simulink model "mrefrobotarm_modified_previous_y_previous_u_previous_ref_Thao"  (R2018b)
settings: Solver=FixedStepAuto  StartTime=0.0  StopTime=10  RelTol=1e-3  AbsTol=1e-6
undefined symbols (not defined in the file or in its folder): sfunxy2
libraries: neural x668, simulink x1
(part 15 of 21)

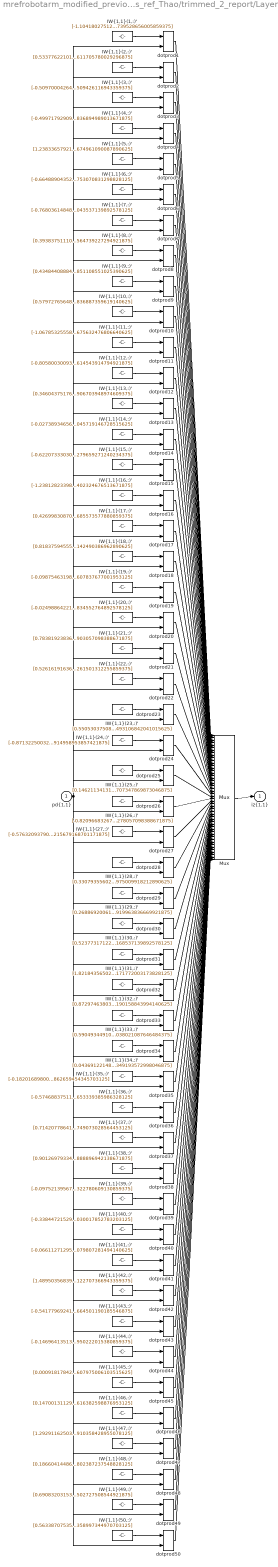
== system mrefrobotarm_modified_previous_y_previous_u_previous_ref_Thao/trimmed_2_report/Layer 1/IW{1,1} ==
  "pd{1,1}" : Inport  PortDimensions=10
      mask Display: e = 0.06;c1 = [120 230 180]/255;c2 = ([120 230 180]+0)/(256+128);c3 = ([120 230 180]+128)/(256+128);patch([0 1 1 0],[0 0 1 1],c1);patch([0 1 1 1-e 1-e 0+e],[0 0 1 1-e 0+e 0+e],c2);patch([0 0 1 1-e 0+e 0+e],[0 1 1 1-e 1-e 0+e],c3);plot([0 1 1 0 0],[0 0 1 1 0]);
  "IW{1,1}(1,:)'" : Constant  Value=[-1.104180275120626220086705870926380157470703125;1.3041448994089861468381741360644809901714324951171875;0.32348674993063841753837550641037523746490478515625;0.0954597345916509965046969909963081590831279754638671875;0.58458283056964244206454850427689962089061737060546875;0.12370355290676347814748936571049853228032588958740234375;-0.360929014481330023844662946430617012083530426025390625;-0.51372399216258501919440959682106040418148040771484375;0.43363839042661889155994003886007703840732574462890625;-0.78302167032477354435826555345556698739528656005859375]
      mask Display: e = 0.06;c1 = [120 150 230]/255;c2 = ([120 150 230]+0)/383;c3 = ([120 150 230]+128)/383;patch([0 1 1 0],[0 0 1 1],c1);patch([0 1 1 1-e 1-e 0+e],[0 0 1 1-e 0+e 0+e],c2);patch([0 0 1 1-e 0+e 0+e],[0 1 1 1-e 1-e 0+e],c3);plot([0 1 1 0 0],[0 0 1 1 0]);disp('Weights');
  "IW{1,1}(10,:)'" : Constant  Value=[0.57972765648551993766801615493022836744785308837890625;0.56702883929374958693614416915806941688060760498046875;0.73417648924284450995259021510719321668148040771484375;-0.545536348624968692178072160459123551845550537109375;-0.85212502298467096562006872773054055869579315185546875;0.9171593407120699481538395048119127750396728515625;0.486441425317741593659093268797732889652252197265625;-1.19193592499658951311403143336065113544464111328125;-0.34835369047706132850095173125737346708774566650390625;-0.277702966436770781744058922413387335836887359619140625]
      mask Display: e = 0.06;c1 = [120 150 230]/255;c2 = ([120 150 230]+0)/383;c3 = ([120 150 230]+128)/383;patch([0 1 1 0],[0 0 1 1],c1);patch([0 1 1 1-e 1-e 0+e],[0 0 1 1-e 0+e 0+e],c2);patch([0 0 1 1-e 0+e 0+e],[0 1 1 1-e 1-e 0+e],c3);plot([0 1 1 0 0],[0 0 1 1 0]);disp('Weights');
  "IW{1,1}(11,:)'" : Constant  Value=[-1.067853255585921257164727649069391191005706787109375;0.73612625892691163631553763480042107403278350830078125;0.6564643621126766692697174221393652260303497314453125;0.2467046979952456087215040270166355185210704803466796875;-0.99137542418344748451630721319816075265407562255859375;-0.265054621061350637045705980199272744357585906982421875;0.086378144705514525725220664753578603267669677734375;-0.5348493447178370718830819896538741886615753173828125;0.3771915850785896306973654645844362676143646240234375;0.617872935716521798354960992583073675632476806640625]
      mask Display: e = 0.06;c1 = [120 150 230]/255;c2 = ([120 150 230]+0)/383;c3 = ([120 150 230]+128)/383;patch([0 1 1 0],[0 0 1 1],c1);patch([0 1 1 1-e 1-e 0+e],[0 0 1 1-e 0+e 0+e],c2);patch([0 0 1 1-e 0+e 0+e],[0 1 1 1-e 1-e 0+e],c3);plot([0 1 1 0 0],[0 0 1 1 0]);disp('Weights');
  "IW{1,1}(12,:)'" : Constant  Value=[-0.80580030093587506900831840539467521011829376220703125;0.76359779607282451951988377913949079811573028564453125;-1.22625268437045331637591516482643783092498779296875;-0.052095597808536391049027969302187557332217693328857421875;-0.65232187763079341191740923022734932601451873779296875;-1.2613588707820095891065648174844682216644287109375;0.48668873664058853734104559407569468021392822265625;0.431726260476050394121472209008061327040195465087890625;-0.98679278575181406107930115467752330005168914794921875;-0.710264778984373901238313919748179614543914794921875]
      mask Display: e = 0.06;c1 = [120 150 230]/255;c2 = ([120 150 230]+0)/383;c3 = ([120 150 230]+128)/383;patch([0 1 1 0],[0 0 1 1],c1);patch([0 1 1 1-e 1-e 0+e],[0 0 1 1-e 0+e 0+e],c2);patch([0 0 1 1-e 0+e 0+e],[0 1 1 1-e 1-e 0+e],c3);plot([0 1 1 0 0],[0 0 1 1 0]);disp('Weights');
  "IW{1,1}(13,:)'" : Constant  Value=[0.34604375176023349780507487594150006771087646484375;0.9479300710749034575286486870027147233486175537109375;-0.1703490730393587837543378782356739975512027740478515625;-0.60778553441507654486741785149206407368183135986328125;0.2485715821018385784935134097395348362624645233154296875;-1.6227947657127679281785503917490132153034210205078125;0.217755149168625428135470656343386508524417877197265625;0.9551408839894250935032005145330913364887237548828125;-0.6000208905664019543024778613471426069736480712890625;-0.266950735484987600187878342694602906703948974609375]
      mask Display: e = 0.06;c1 = [120 150 230]/255;c2 = ([120 150 230]+0)/383;c3 = ([120 150 230]+128)/383;patch([0 1 1 0],[0 0 1 1],c1);patch([0 1 1 1-e 1-e 0+e],[0 0 1 1-e 0+e 0+e],c2);patch([0 0 1 1-e 0+e 0+e],[0 1 1 1-e 1-e 0+e],c3);plot([0 1 1 0 0],[0 0 1 1 0]);disp('Weights');
  "IW{1,1}(14,:)'" : Constant  Value=[-0.0273893465600874193299762993092372198589146137237548828125;-0.41727030088538763497041372829698957502841949462890625;-0.0236305029994381132762981678752112202346324920654296875;0.99142437831494600875004152840119786560535430908203125;-0.606387468788796457630496661295183002948760986328125;0.644974946776212476606815471313893795013427734375;1.15494261537616349500012802309356629848480224609375;0.147283871931444598768479181671864353120326995849609375;1.144113546152838889469194327830336987972259521484375;-0.0650154200029232909319176769713521935045719146728515625]
      mask Display: e = 0.06;c1 = [120 150 230]/255;c2 = ([120 150 230]+0)/383;c3 = ([120 150 230]+128)/383;patch([0 1 1 0],[0 0 1 1],c1);patch([0 1 1 1-e 1-e 0+e],[0 0 1 1-e 0+e 0+e],c2);patch([0 0 1 1-e 0+e 0+e],[0 1 1 1-e 1-e 0+e],c3);plot([0 1 1 0 0],[0 0 1 1 0]);disp('Weights');
  "IW{1,1}(15,:)'" : Constant  Value=[-0.62207333030785683103403016502852551639080047607421875;0.1991080763831607203240281478429096750915050506591796875;-0.1321839786478450073925472452174290083348751068115234375;0.0036825292739893172692944300905537602375261485576629638671875;-0.64224566379800485105278085029567591845989227294921875;-1.4376578529579646659186664692242629826068878173828125;-0.3079825786544854171467022752040065824985504150390625;-0.206732957747276457904916924235294573009014129638671875;1.210694115781494328842882168828509747982025146484375;0.61406110053037943341536220032139681279659271240234375]
      mask Display: e = 0.06;c1 = [120 150 230]/255;c2 = ([120 150 230]+0)/383;c3 = ([120 150 230]+128)/383;patch([0 1 1 0],[0 0 1 1],c1);patch([0 1 1 1-e 1-e 0+e],[0 0 1 1-e 0+e 0+e],c2);patch([0 0 1 1-e 0+e 0+e],[0 1 1 1-e 1-e 0+e],c3);plot([0 1 1 0 0],[0 0 1 1 0]);disp('Weights');
  "IW{1,1}(16,:)'" : Constant  Value=[-1.238128233985433812591736568720079958438873291015625;2.3065545792792594426146024488843977451324462890625;0.364870321916919093663267403826466761529445648193359375;1.2422644219105254403956450914847664535045623779296875;1.3947104860949135485270744538865983486175537109375;-1.1075435848184638221169961980194784700870513916015625;-1.097263923921735884192685261950828135013580322265625;1.2626135619126628295560976766864769160747528076171875;1.4728383027981932773542439463199116289615631103515625;-0.282194300572370604385241676936857402324676513671875]
      mask Display: e = 0.06;c1 = [120 150 230]/255;c2 = ([120 150 230]+0)/383;c3 = ([120 150 230]+128)/383;patch([0 1 1 0],[0 0 1 1],c1);patch([0 1 1 1-e 1-e 0+e],[0 0 1 1-e 0+e 0+e],c2);patch([0 0 1 1-e 0+e 0+e],[0 1 1 1-e 1-e 0+e],c3);plot([0 1 1 0 0],[0 0 1 1 0]);disp('Weights');
  "IW{1,1}(17,:)'" : Constant  Value=[0.4269983087004598498737095724209211766719818115234375;0.53358524841212096045950374900712631642818450927734375;-0.889948604603941983981485464028082787990570068359375;0.360282648313135667184070598523248918354511260986328125;0.59479992088535460492693118794704787433147430419921875;-0.3772952231089867769497914196108467876911163330078125;0.16556798383700621624115001395693980157375335693359375;-0.8744182056579965500731077554519288241863250732421875;0.3655577086366708083886578606325201690196990966796875;0.752955685864106438742737736902199685573577880859375]
      mask Display: e = 0.06;c1 = [120 150 230]/255;c2 = ([120 150 230]+0)/383;c3 = ([120 150 230]+128)/383;patch([0 1 1 0],[0 0 1 1],c1);patch([0 1 1 1-e 1-e 0+e],[0 0 1 1-e 0+e 0+e],c2);patch([0 0 1 1-e 0+e 0+e],[0 1 1 1-e 1-e 0+e],c3);plot([0 1 1 0 0],[0 0 1 1 0]);disp('Weights');
  "IW{1,1}(18,:)'" : Constant  Value=[0.8183759455560257745077024083002470433712005615234375;-0.89419721912882932368660249267122708261013031005859375;-0.04029197370486048423998681755620054900646209716796875;-0.7316325646520580594511784511269070208072662353515625;1.3309392300203446435347132137394510209560394287109375;0.7753645817321903610519484573160298168659210205078125;0.002863573304035552276325393705747046624310314655303955078125;0.0115718294676535916887250010631760233081877231597900390625;-0.09187746511239069935328416249831207096576690673828125;0.048058113968365880064315120989704155363142490386962890625]
      mask Display: e = 0.06;c1 = [120 150 230]/255;c2 = ([120 150 230]+0)/383;c3 = ([120 150 230]+128)/383;patch([0 1 1 0],[0 0 1 1],c1);patch([0 1 1 1-e 1-e 0+e],[0 0 1 1-e 0+e 0+e],c2);patch([0 0 1 1-e 0+e 0+e],[0 1 1 1-e 1-e 0+e],c3);plot([0 1 1 0 0],[0 0 1 1 0]);disp('Weights');
  "IW{1,1}(19,:)'" : Constant  Value=[-0.0987546319835528318975548245362006127834320068359375;0.6081607495239078620130612762295641005039215087890625;0.65858352740219039400670908435131423175334930419921875;-0.901487079776840172229412928572855889797210693359375;0.820869730694437027551657592994160950183868408203125;-0.061664555689623902490215101579451584257185459136962890625;-0.06555393878289837716888399654635577462613582611083984375;-0.39833146139729425083686464859056286513805389404296875;0.202125799001910133601001007264130748808383941650390625;-0.97060645735931505573290678512421436607837677001953125]
      mask Display: e = 0.06;c1 = [120 150 230]/255;c2 = ([120 150 230]+0)/383;c3 = ([120 150 230]+128)/383;patch([0 1 1 0],[0 0 1 1],c1);patch([0 1 1 1-e 1-e 0+e],[0 0 1 1-e 0+e 0+e],c2);patch([0 0 1 1-e 0+e 0+e],[0 1 1 1-e 1-e 0+e],c3);plot([0 1 1 0 0],[0 0 1 1 0]);disp('Weights');
  "IW{1,1}(2,:)'" : Constant  Value=[0.533776221018695817832622196874581277370452880859375;0.1819770919475681425492297194068669341504573822021484375;-1.7509652530362231903637848517973907291889190673828125;0.3054714691309958762843734803027473390102386474609375;-0.6380191897078579810198561972356401383876800537109375;-0.1946898637866417980379907248789095319807529449462890625;0.420775402616209326378537980417604558169841766357421875;1.1041430408562578069364690236398018896579742431640625;-0.176572820691475007581772160847322084009647369384765625;0.88087433619841337684164273014175705611705780029296875]
      mask Display: e = 0.06;c1 = [120 150 230]/255;c2 = ([120 150 230]+0)/383;c3 = ([120 150 230]+128)/383;patch([0 1 1 0],[0 0 1 1],c1);patch([0 1 1 1-e 1-e 0+e],[0 0 1 1-e 0+e 0+e],c2);patch([0 0 1 1-e 0+e 0+e],[0 1 1 1-e 1-e 0+e],c3);plot([0 1 1 0 0],[0 0 1 1 0]);disp('Weights');
  "IW{1,1}(20,:)'" : Constant  Value=[-0.0249886422195137736235182046584668569266796112060546875;-1.3838462156369286670809515271685086190700531005859375;0.83011337269990115306228517511044628918170928955078125;-0.71273621772459672119026663494878448545932769775390625;-0.984316911842150421563246709411032497882843017578125;0.2501542837986285849893874910776503384113311767578125;-0.295607634991452983275195265377988107502460479736328125;-0.387214543407977895839167103986255824565887451171875;-0.1931330822692971793674843183907796628773212432861328125;-0.56906603587908854979815487240557558834552764892578125]
      mask Display: e = 0.06;c1 = [120 150 230]/255;c2 = ([120 150 230]+0)/383;c3 = ([120 150 230]+128)/383;patch([0 1 1 0],[0 0 1 1],c1);patch([0 1 1 1-e 1-e 0+e],[0 0 1 1-e 0+e 0+e],c2);patch([0 0 1 1-e 0+e 0+e],[0 1 1 1-e 1-e 0+e],c3);plot([0 1 1 0 0],[0 0 1 1 0]);disp('Weights');
  "IW{1,1}(21,:)'" : Constant  Value=[0.78381923836040201525321435838122852146625518798828125;-0.44474514989193958403035367155098356306552886962890625;0.0983399806929019515422396580106578767299652099609375;1.003408964396794278428615143639035522937774658203125;-0.652345075278432329213273987988941371440887451171875;0.328319503237768650638628287197207100689411163330078125;-1.1488063518367983562029621680267155170440673828125;-0.1647676740851701515655491903089568950235843658447265625;0.7494815823502161133973231699201278388500213623046875;-0.29854112680218036768309275430510751903057098388671875]
      mask Display: e = 0.06;c1 = [120 150 230]/255;c2 = ([120 150 230]+0)/383;c3 = ([120 150 230]+128)/383;patch([0 1 1 0],[0 0 1 1],c1);patch([0 1 1 1-e 1-e 0+e],[0 0 1 1-e 0+e 0+e],c2);patch([0 0 1 1-e 0+e 0+e],[0 1 1 1-e 1-e 0+e],c3);plot([0 1 1 0 0],[0 0 1 1 0]);disp('Weights');
  "IW{1,1}(22,:)'" : Constant  Value=[0.5261619163611890304110829674755223095417022705078125;1.4484359314933870077624078476219438016414642333984375;0.86231124186971908063270575439673848450183868408203125;-0.973829112303234101233329056412912905216217041015625;1.7443507343296100753349264778080396354198455810546875;-0.81708725256885694765429661856614984571933746337890625;-0.63383422742480222122907207449316047132015228271484375;-0.48168645915917085442714551390963606536388397216796875;-0.57070797609170476061279941859538666903972625732421875;1.0879276870040468505607123006484471261501312255859375]
      mask Display: e = 0.06;c1 = [120 150 230]/255;c2 = ([120 150 230]+0)/383;c3 = ([120 150 230]+128)/383;patch([0 1 1 0],[0 0 1 1],c1);patch([0 1 1 1-e 1-e 0+e],[0 0 1 1-e 0+e 0+e],c2);patch([0 0 1 1-e 0+e 0+e],[0 1 1 1-e 1-e 0+e],c3);plot([0 1 1 0 0],[0 0 1 1 0]);disp('Weights');
  "IW{1,1}(23,:)'" : Constant  Value=[0.550530375086509149440416877041570842266082763671875;-0.397862366630399921785254946371424011886119842529296875;0.2039531605920501533546485006809234619140625;-0.92412252569438246840860529118799604475498199462890625;-0.094079798965390371012773584880051203072071075439453125;-1.388821073650537751831279820180498063564300537109375;-0.327663280010716706502904571607359685003757476806640625;0.25884295164939175037943641655147075653076171875;0.316577252595158231684990823850966989994049072265625;0.688439495772796394845727263600565493106842041015625]
      mask Display: e = 0.06;c1 = [120 150 230]/255;c2 = ([120 150 230]+0)/383;c3 = ([120 150 230]+128)/383;patch([0 1 1 0],[0 0 1 1],c1);patch([0 1 1 1-e 1-e 0+e],[0 0 1 1-e 0+e 0+e],c2);patch([0 0 1 1-e 0+e 0+e],[0 1 1 1-e 1-e 0+e],c3);plot([0 1 1 0 0],[0 0 1 1 0]);disp('Weights');
  "IW{1,1}(24,:)'" : Constant  Value=[-0.87132250032686930918401913004345260560512542724609375;-0.26328418798328068195502282833331264555454254150390625;0.99061115791988729739614427671767771244049072265625;-0.398616888955526604831902659498155117034912109375;1.5531789047066297815291591177810914814472198486328125;-1.1031450574578502976663685331004671752452850341796875;0.0650202718377247690373366140192956663668155670166015625;-0.03086656480857978557263976426838780753314495086669921875;-0.44995060413095888662837751326151192188262939453125;1.9713467333387562074875631878967396914958953857421875]
      mask Display: e = 0.06;c1 = [120 150 230]/255;c2 = ([120 150 230]+0)/383;c3 = ([120 150 230]+128)/383;patch([0 1 1 0],[0 0 1 1],c1);patch([0 1 1 1-e 1-e 0+e],[0 0 1 1-e 0+e 0+e],c2);patch([0 0 1 1-e 0+e 0+e],[0 1 1 1-e 1-e 0+e],c3);plot([0 1 1 0 0],[0 0 1 1 0]);disp('Weights');
  "IW{1,1}(25,:)'" : Constant  Value=[0.1462113413166806485943283178130513988435268402099609375;-0.5010328728309134671548008554964326322078704833984375;-0.38307558363141314128341718969750218093395233154296875;-0.0001930945276350111948493459834708119160495698451995849609375;0.6996439098394995337315549477352760732173919677734375;0.97088905712405637604689445652184076607227325439453125;0.26430527893956201612724044025526382029056549072265625;-1.402165562910202556423655551043339073657989501953125;0.97619757519551864088924730822327546775341033935546875;-1.4487075930507440357786208551260642707347869873046875]
      mask Display: e = 0.06;c1 = [120 150 230]/255;c2 = ([120 150 230]+0)/383;c3 = ([120 150 230]+128)/383;patch([0 1 1 0],[0 0 1 1],c1);patch([0 1 1 1-e 1-e 0+e],[0 0 1 1-e 0+e 0+e],c2);patch([0 0 1 1-e 0+e 0+e],[0 1 1 1-e 1-e 0+e],c3);plot([0 1 1 0 0],[0 0 1 1 0]);disp('Weights');
  "IW{1,1}(26,:)'" : Constant  Value=[-0.820966832675215751891073523438535630702972412109375;-1.0042969558633221272003765989211387932300567626953125;0.75291819339959176193843859437038190662860870361328125;-0.84829588157059176989349680297891609370708465576171875;-0.87836311429813063167415521093062125146389007568359375;-0.211503334542910703675033801118843257427215576171875;-1.0003829781543329691118060509325005114078521728515625;-0.47554127174002125411078623073990456759929656982421875;-1.030992482353195516253663299721665680408477783203125;-0.92349222552234788707892221282236278057098388671875]
      mask Display: e = 0.06;c1 = [120 150 230]/255;c2 = ([120 150 230]+0)/383;c3 = ([120 150 230]+128)/383;patch([0 1 1 0],[0 0 1 1],c1);patch([0 1 1 1-e 1-e 0+e],[0 0 1 1-e 0+e 0+e],c2);patch([0 0 1 1-e 0+e 0+e],[0 1 1 1-e 1-e 0+e],c3);plot([0 1 1 0 0],[0 0 1 1 0]);disp('Weights');
  "IW{1,1}(27,:)'" : Constant  Value=[-0.57632093790316385462091375302406959235668182373046875;-0.35565547080635406818061028388910926878452301025390625;1.334695428313806164766219808370806276798248291015625;-0.82448708081768640187902974503231234848499298095703125;-0.195651938678662540294084237757488153874874114990234375;0.5328672554072977352035422882181592285633087158203125;-0.909222111031680046977498932392336428165435791015625;-0.2241048337298519876892299862447544001042842864990234375;0.1575311858593370917258624785972642712295055389404296875;0.062733318523321812687498777449945919215679168701171875]
      mask Display: e = 0.06;c1 = [120 150 230]/255;c2 = ([120 150 230]+0)/383;c3 = ([120 150 230]+128)/383;patch([0 1 1 0],[0 0 1 1],c1);patch([0 1 1 1-e 1-e 0+e],[0 0 1 1-e 0+e 0+e],c2);patch([0 0 1 1-e 0+e 0+e],[0 1 1 1-e 1-e 0+e],c3);plot([0 1 1 0 0],[0 0 1 1 0]);disp('Weights');
  "IW{1,1}(28,:)'" : Constant  Value=[0.3307935560220418569343792114523239433765411376953125;-0.55113396576540207849603802969795651733875274658203125;0.569175453393025776449576369486749172210693359375;1.0623796197910062577562939623021520674228668212890625;1.01352180940139202647287675063125789165496826171875;0.6277889800107125939376828682725317776203155517578125;0.509005323293744371682123528444208204746246337890625;0.182846956508069868885257847068714909255504608154296875;-0.9376417446073606054568472245591692626476287841796875;-0.453358199464616584695164647200726903975009918212890625]
      mask Display: e = 0.06;c1 = [120 150 230]/255;c2 = ([120 150 230]+0)/383;c3 = ([120 150 230]+128)/383;patch([0 1 1 0],[0 0 1 1],c1);patch([0 1 1 1-e 1-e 0+e],[0 0 1 1-e 0+e 0+e],c2);patch([0 0 1 1-e 0+e 0+e],[0 1 1 1-e 1-e 0+e],c3);plot([0 1 1 0 0],[0 0 1 1 0]);disp('Weights');
  "IW{1,1}(29,:)'" : Constant  Value=[0.2688692006136645940017615430406294763088226318359375;-0.185266062760000294051820901586324907839298248291015625;-0.9934232787889960558658231093431822955608367919921875;-0.85017036952777313985052387579344213008880615234375;0.8797380692364245025061109117814339697360992431640625;-0.57780560479178377786269038551836274564266204833984375;0.152556349829305271104118446601205505430698394775390625;0.042106754659083346636894162884345860220491886138916015625;0.2277901161133095431221562421342241577804088592529296875;-0.6136323086632990975175516723538748919963836669921875]
      mask Display: e = 0.06;c1 = [120 150 230]/255;c2 = ([120 150 230]+0)/383;c3 = ([120 150 230]+128)/383;patch([0 1 1 0],[0 0 1 1],c1);patch([0 1 1 1-e 1-e 0+e],[0 0 1 1-e 0+e 0+e],c2);patch([0 0 1 1-e 0+e 0+e],[0 1 1 1-e 1-e 0+e],c3);plot([0 1 1 0 0],[0 0 1 1 0]);disp('Weights');
  "IW{1,1}(3,:)'" : Constant  Value=[-0.50970004264338963917424507599207572638988494873046875;0.06751525411120228026273792920619598589837551116943359375;-0.34641617332988705602048185028252191841602325439453125;0.9385874812029564306925522032543085515499114990234375;-0.2054274924435462723604217671891092322766780853271484375;0.320125171249427020736533222589059732854366302490234375;0.63030949671083547070082886421005241572856903076171875;-0.2298860542419578767425747400920954532921314239501953125;-0.98055941667693746754963513012626208364963531494140625;1.2646827500011139644442437202087603509426116943359375]
      mask Display: e = 0.06;c1 = [120 150 230]/255;c2 = ([120 150 230]+0)/383;c3 = ([120 150 230]+128)/383;patch([0 1 1 0],[0 0 1 1],c1);patch([0 1 1 1-e 1-e 0+e],[0 0 1 1-e 0+e 0+e],c2);patch([0 0 1 1-e 0+e 0+e],[0 1 1 1-e 1-e 0+e],c3);plot([0 1 1 0 0],[0 0 1 1 0]);disp('Weights');
  "IW{1,1}(30,:)'" : Constant  Value=[0.52377317122200517385266493874951265752315521240234375;-0.61899210000905735551413044959190301597118377685546875;0.28879624708624629381148452011984772980213165283203125;0.94336102880949856963610500315553508698940277099609375;0.84545222899391470061658537815674208104610443115234375;-0.75153431922312952107034789150930009782314300537109375;-0.5674167894000470280246872789575718343257904052734375;-0.6827513389171018243217758936225436627864837646484375;-0.6337361889801311765069158354890532791614532470703125;-0.7930113257051722985835340296034701168537139892578125]
      mask Display: e = 0.06;c1 = [120 150 230]/255;c2 = ([120 150 230]+0)/383;c3 = ([120 150 230]+128)/383;patch([0 1 1 0],[0 0 1 1],c1);patch([0 1 1 1-e 1-e 0+e],[0 0 1 1-e 0+e 0+e],c2);patch([0 0 1 1-e 0+e 0+e],[0 1 1 1-e 1-e 0+e],c3);plot([0 1 1 0 0],[0 0 1 1 0]);disp('Weights');
  "IW{1,1}(31,:)'" : Constant  Value=[1.8218435650275648374218917524558492004871368408203125;-0.58117478360756102961914848492597229778766632080078125;-0.6218791097566243042393807627377100288867950439453125;0.38029716104421351641207138527533970773220062255859375;-0.650416961899480838837916962802410125732421875;0.79032592458809602931069093756377696990966796875;0.89640949591250052019830718563753180205821990966796875;0.472770437947413080248537653460516594350337982177734375;0.2160992616503935870309049960269476287066936492919921875;0.73238617773512360020760070256073959171772003173828125]
      mask Display: e = 0.06;c1 = [120 150 230]/255;c2 = ([120 150 230]+0)/383;c3 = ([120 150 230]+128)/383;patch([0 1 1 0],[0 0 1 1],c1);patch([0 1 1 1-e 1-e 0+e],[0 0 1 1-e 0+e 0+e],c2);patch([0 0 1 1-e 0+e 0+e],[0 1 1 1-e 1-e 0+e],c3);plot([0 1 1 0 0],[0 0 1 1 0]);disp('Weights');
  "IW{1,1}(32,:)'" : Constant  Value=[0.872974638033729544162042657262645661830902099609375;-0.09320475893425396451963393928963341750204563140869140625;-1.03298686444966580921800414216704666614532470703125;0.8491159515026069914966910801013000309467315673828125;-0.9267004738023183474382449276163242757320404052734375;0.8781581312669437533457994504715315997600555419921875;0.483922895302127564765015677039627917110919952392578125;-0.5433128137878793229020857324940152466297149658203125;1.44038756703261672242888380424119532108306884765625;0.272188910568918418508843615200021304190158843994140625]
      mask Display: e = 0.06;c1 = [120 150 230]/255;c2 = ([120 150 230]+0)/383;c3 = ([120 150 230]+128)/383;patch([0 1 1 0],[0 0 1 1],c1);patch([0 1 1 1-e 1-e 0+e],[0 0 1 1-e 0+e 0+e],c2);patch([0 0 1 1-e 0+e 0+e],[0 1 1 1-e 1-e 0+e],c3);plot([0 1 1 0 0],[0 0 1 1 0]);disp('Weights');
  "IW{1,1}(33,:)'" : Constant  Value=[0.5904934491003765995031926649971865117549896240234375;-0.126961369115498212689630008753738366067409515380859375;-1.037275508881108532222015128354541957378387451171875;0.3334712650241133946593663495150394737720489501953125;-1.315873881733157002571488192188553512096405029296875;-0.77271696951212864856728401719010435044765472412109375;-0.4789712009451128071901848670677281916141510009765625;-0.314439066697734859179291788677801378071308135986328125;-1.4540645478785505506635900019318796694278717041015625;-0.2234591610915442616569492884082137607038021087646484375]
      mask Display: e = 0.06;c1 = [120 150 230]/255;c2 = ([120 150 230]+0)/383;c3 = ([120 150 230]+128)/383;patch([0 1 1 0],[0 0 1 1],c1);patch([0 1 1 1-e 1-e 0+e],[0 0 1 1-e 0+e 0+e],c2);patch([0 0 1 1-e 0+e 0+e],[0 1 1 1-e 1-e 0+e],c3);plot([0 1 1 0 0],[0 0 1 1 0]);disp('Weights');
  "IW{1,1}(34,:)'" : Constant  Value=[0.043691221483490853827458266778194229118525981903076171875;0.425702588003492865542654044475057162344455718994140625;0.167425942290460538774965471020550467073917388916015625;-0.6288326384348434938686978057376109063625335693359375;-0.63305584322113828132927437764010392129421234130859375;0.1555373693786098188152067223199992440640926361083984375;-0.2209460532163330104271636855628457851707935333251953125;0.392438370463115415720523060372215695679187774658203125;0.1683507980273061532816569751958013512194156646728515625;0.8691052880575422801001650441321544349193572998046875]
      mask Display: e = 0.06;c1 = [120 150 230]/255;c2 = ([120 150 230]+0)/383;c3 = ([120 150 230]+128)/383;patch([0 1 1 0],[0 0 1 1],c1);patch([0 1 1 1-e 1-e 0+e],[0 0 1 1-e 0+e 0+e],c2);patch([0 0 1 1-e 0+e 0+e],[0 1 1 1-e 1-e 0+e],c3);plot([0 1 1 0 0],[0 0 1 1 0]);disp('Weights');
  "IW{1,1}(35,:)'" : Constant  Value=[-0.1820168980060662689002271008575917221605777740478515625;-0.5619071320381916478936545900069177150726318359375;-0.267364968221916299295770613753120414912700653076171875;-0.52280083522110920579706316857482306659221649169921875;0.424125790881571484991496845395886339247226715087890625;0.0009256708429006333706257070303990985848940908908843994140625;-1.0041230495716770843017684455844573676586151123046875;-0.77601669041627296952157166742836125195026397705078125;0.0436137270972177526484614418222918175160884857177734375;-1.2403815101047481750384804399800486862659454345703125]
      mask Display: e = 0.06;c1 = [120 150 230]/255;c2 = ([120 150 230]+0)/383;c3 = ([120 150 230]+128)/383;patch([0 1 1 0],[0 0 1 1],c1);patch([0 1 1 1-e 1-e 0+e],[0 0 1 1-e 0+e 0+e],c2);patch([0 0 1 1-e 0+e 0+e],[0 1 1 1-e 1-e 0+e],c3);plot([0 1 1 0 0],[0 0 1 1 0]);disp('Weights');
  "IW{1,1}(36,:)'" : Constant  Value=[-0.5746883751172446874733168442617170512676239013671875;-0.03739487089902081284886747880591428838670253753662109375;0.2829041056481056415350394672714173793792724609375;0.455025978207705905642654897746979258954524993896484375;0.56596631934457519719217089004814624786376953125;-0.60637750846840232643586432459414936602115631103515625;-0.87072297195806258596206816946505568921566009521484375;1.01716310962299605336056629312224686145782470703125;0.74535601968146247831015216434025205671787261962890625;0.4989297079723826744412917832960374653339385986328125]
      mask Display: e = 0.06;c1 = [120 150 230]/255;c2 = ([120 150 230]+0)/383;c3 = ([120 150 230]+128)/383;patch([0 1 1 0],[0 0 1 1],c1);patch([0 1 1 1-e 1-e 0+e],[0 0 1 1-e 0+e 0+e],c2);patch([0 0 1 1-e 0+e 0+e],[0 1 1 1-e 1-e 0+e],c3);plot([0 1 1 0 0],[0 0 1 1 0]);disp('Weights');
  "IW{1,1}(37,:)'" : Constant  Value=[0.71420778641449922385930904056294821202754974365234375;0.100736969441503732003440063635935075581073760986328125;0.9823970523319036640685908423620276153087615966796875;0.41265551251273435706679038048605434596538543701171875;1.0348771920462735973700318936607800424098968505859375;1.13678417226512440407759640947915613651275634765625;0.2067039297753831827986203961700084619224071502685546875;-0.89199831226248615934082408784888684749603271484375;0.31491113509433599215725507747265510261058807373046875;-0.465383020462850016674138942107674665749073028564453125]
      mask Display: e = 0.06;c1 = [120 150 230]/255;c2 = ([120 150 230]+0)/383;c3 = ([120 150 230]+128)/383;patch([0 1 1 0],[0 0 1 1],c1);patch([0 1 1 1-e 1-e 0+e],[0 0 1 1-e 0+e 0+e],c2);patch([0 0 1 1-e 0+e 0+e],[0 1 1 1-e 1-e 0+e],c3);plot([0 1 1 0 0],[0 0 1 1 0]);disp('Weights');
  "IW{1,1}(38,:)'" : Constant  Value=[0.9012697933448714504578447304083965718746185302734375;-0.57092470713486764832822473181295208632946014404296875;-0.6664381112183501709722577288630418479442596435546875;0.3935606287085418042437368058017455041408538818359375;-1.143883802769684709943476264015771448612213134765625;-0.53101573932611556561056431746692396700382232666015625;-0.283373205006573147812787283328361809253692626953125;0.5118696330561556262495059854700230062007904052734375;1.0550573165964640676151020670658908784389495849609375;-0.2957771856839002122541160133550874888896942138671875]
      mask Display: e = 0.06;c1 = [120 150 230]/255;c2 = ([120 150 230]+0)/383;c3 = ([120 150 230]+128)/383;patch([0 1 1 0],[0 0 1 1],c1);patch([0 1 1 1-e 1-e 0+e],[0 0 1 1-e 0+e 0+e],c2);patch([0 0 1 1-e 0+e 0+e],[0 1 1 1-e 1-e 0+e],c3);plot([0 1 1 0 0],[0 0 1 1 0]);disp('Weights');
  "IW{1,1}(39,:)'" : Constant  Value=[-0.09752139567874414105563829480161075480282306671142578125;-1.654997221988329325625954879797063767910003662109375;-0.441968574709696027102978632683516480028629302978515625;-1.2901490836893987346201129184919409453868865966796875;0.28124999593129584862793990396312437951564788818359375;0.329188037856861459573565298342145979404449462890625;-0.98218391549703654153091747502912767231464385986328125;0.470799228030611416340178720929543487727642059326171875;-0.73725750644395449118206897765048779547214508056640625;-0.293558789566588484998277408521971665322780609130859375]
      mask Display: e = 0.06;c1 = [120 150 230]/255;c2 = ([120 150 230]+0)/383;c3 = ([120 150 230]+128)/383;patch([0 1 1 0],[0 0 1 1],c1);patch([0 1 1 1-e 1-e 0+e],[0 0 1 1-e 0+e 0+e],c2);patch([0 0 1 1-e 0+e 0+e],[0 1 1 1-e 1-e 0+e],c3);plot([0 1 1 0 0],[0 0 1 1 0]);disp('Weights');
  "IW{1,1}(4,:)'" : Constant  Value=[-0.49971792909020684714249682656372897326946258544921875;0.2451619575692929042798340333320084027945995330810546875;-0.10554499894506079449296720440543140284717082977294921875;1.05357291761016114151061628945171833038330078125;-0.7244168776944792664806982429581694304943084716796875;0.51827510388793018858422101402538828551769256591796875;-0.321138581780947507393619844151544384658336639404296875;-0.19493532473627495082979521612287499010562896728515625;0.2136768776370955025267761584473191760480403900146484375;-1.612407001173789211634357343427836894989013671875]
      mask Display: e = 0.06;c1 = [120 150 230]/255;c2 = ([120 150 230]+0)/383;c3 = ([120 150 230]+128)/383;patch([0 1 1 0],[0 0 1 1],c1);patch([0 1 1 1-e 1-e 0+e],[0 0 1 1-e 0+e 0+e],c2);patch([0 0 1 1-e 0+e 0+e],[0 1 1 1-e 1-e 0+e],c3);plot([0 1 1 0 0],[0 0 1 1 0]);disp('Weights');
  "IW{1,1}(40,:)'" : Constant  Value=[-0.338447215294792880246887989414972253143787384033203125;1.145666269260541270114117651246488094329833984375;1.043032887989355561586535259266383945941925048828125;0.965335232740152537900257811998017132282257080078125;-0.78507152208093955447765210919897072017192840576171875;-0.68485339577537540645124636284890584647655487060546875;0.40023872879740685082339268774376250803470611572265625;-0.36857013326388010643341885952395386993885040283203125;0.30053800572688904590989977805293165147304534912109375;-0.4236535184979157708795582948368974030017852783203125]
      mask Display: e = 0.06;c1 = [120 150 230]/255;c2 = ([120 150 230]+0)/383;c3 = ([120 150 230]+128)/383;patch([0 1 1 0],[0 0 1 1],c1);patch([0 1 1 1-e 1-e 0+e],[0 0 1 1-e 0+e 0+e],c2);patch([0 0 1 1-e 0+e 0+e],[0 1 1 1-e 1-e 0+e],c3);plot([0 1 1 0 0],[0 0 1 1 0]);disp('Weights');
  "IW{1,1}(41,:)'" : Constant  Value=[-0.06611271295832299443873125710524618625640869140625;0.1757436784119395800640717197893536649644374847412109375;1.0324431692368347679433782104752026498317718505859375;-1.0626353505992012227210352648398838937282562255859375;-1.268986870164570124330793987610377371311187744140625;-0.329384428901188408556066633536829613149166107177734375;-1.2351667211580086291888846972142346203327178955078125;-0.72422070826349427274948311605839990079402923583984375;0.64332056813114224524952078354544937610626220703125;-0.1355095270701160148352215628619887866079807281494140625]
      mask Display: e = 0.06;c1 = [120 150 230]/255;c2 = ([120 150 230]+0)/383;c3 = ([120 150 230]+128)/383;patch([0 1 1 0],[0 0 1 1],c1);patch([0 1 1 1-e 1-e 0+e],[0 0 1 1-e 0+e 0+e],c2);patch([0 0 1 1-e 0+e 0+e],[0 1 1 1-e 1-e 0+e],c3);plot([0 1 1 0 0],[0 0 1 1 0]);disp('Weights');
  "IW{1,1}(42,:)'" : Constant  Value=[1.4895035683919133351338359716464765369892120361328125;-0.407532311135206215535475848810165189206600189208984375;-0.48555676048555074242329965272801928222179412841796875;-0.09141304491246203534071668173055513761937618255615234375;0.349377834424366484622481721089570783078670501708984375;-0.413265070859394623159488446617615409195423126220703125;0.61150929335987458390633264571079052984714508056640625;-0.8457486363201611734297102884738706052303314208984375;0.485089577584606190807647863039164803922176361083984375;-0.194065568689795353574112368733040057122707366943359375]
      mask Display: e = 0.06;c1 = [120 150 230]/255;c2 = ([120 150 230]+0)/383;c3 = ([120 150 230]+128)/383;patch([0 1 1 0],[0 0 1 1],c1);patch([0 1 1 1-e 1-e 0+e],[0 0 1 1-e 0+e 0+e],c2);patch([0 0 1 1-e 0+e 0+e],[0 1 1 1-e 1-e 0+e],c3);plot([0 1 1 0 0],[0 0 1 1 0]);disp('Weights');
  "IW{1,1}(43,:)'" : Constant  Value=[-0.54177969241274126499519070421229116618633270263671875;-0.98299945439460945095788702019490301609039306640625;-0.58507438407505663047203370297211222350597381591796875;-0.57373463395423651700610889747622422873973846435546875;-1.113081709690256548839215611224062740802764892578125;0.60014902904523381721446639858186244964599609375;0.344065815803955177276662880103685893118381500244140625;0.17664632406017977128698248634464107453823089599609375;-1.1046223889388071537354107931605540215969085693359375;-0.2166065764324296150089566026508691720664501190185546875]
      mask Display: e = 0.06;c1 = [120 150 230]/255;c2 = ([120 150 230]+0)/383;c3 = ([120 150 230]+128)/383;patch([0 1 1 0],[0 0 1 1],c1);patch([0 1 1 1-e 1-e 0+e],[0 0 1 1-e 0+e 0+e],c2);patch([0 0 1 1-e 0+e 0+e],[0 1 1 1-e 1-e 0+e],c3);plot([0 1 1 0 0],[0 0 1 1 0]);disp('Weights');
  "IW{1,1}(44,:)'" : Constant  Value=[-0.1469641351312080956859063007868826389312744140625;-0.63803129205809849811004141884041018784046173095703125;-0.59295554580684528556133727761334739625453948974609375;0.059632722627935196013648777579874149523675441741943359375;-0.69484534699060829243677517297328449785709381103515625;-0.8685744026061736899890775021049194037914276123046875;-1.0013576661169223402936268030316568911075592041015625;0.250268410694419241036001722022774629294872283935546875;-0.98882161586115824292164688813500106334686279296875;0.28676935316048923763077027615508995950222015380859375]
      mask Display: e = 0.06;c1 = [120 150 230]/255;c2 = ([120 150 230]+0)/383;c3 = ([120 150 230]+128)/383;patch([0 1 1 0],[0 0 1 1],c1);patch([0 1 1 1-e 1-e 0+e],[0 0 1 1-e 0+e 0+e],c2);patch([0 0 1 1-e 0+e 0+e],[0 1 1 1-e 1-e 0+e],c3);plot([0 1 1 0 0],[0 0 1 1 0]);disp('Weights');
  "IW{1,1}(45,:)'" : Constant  Value=[0.000918178421387516314859655874869304170715622603893280029296875;0.351223405889607376284544670852483250200748443603515625;-0.60775209219079207034752698746160604059696197509765625;0.88476038910003829141004416669602505862712860107421875;1.5657172805632086909355393800069577991962432861328125;0.03073907922654217639291118757682852447032928466796875;-0.76188039353307879242294120558653958141803741455078125;-0.2150262467881601524677392944795428775250911712646484375;-0.1948121857554230285103358255582861602306365966796875;1.32518243871324248317478122771717607975006103515625]
      mask Display: e = 0.06;c1 = [120 150 230]/255;c2 = ([120 150 230]+0)/383;c3 = ([120 150 230]+128)/383;patch([0 1 1 0],[0 0 1 1],c1);patch([0 1 1 1-e 1-e 0+e],[0 0 1 1-e 0+e 0+e],c2);patch([0 0 1 1-e 0+e 0+e],[0 1 1 1-e 1-e 0+e],c3);plot([0 1 1 0 0],[0 0 1 1 0]);disp('Weights');
  "IW{1,1}(46,:)'" : Constant  Value=[0.1470013112914851094448209778420277871191501617431640625;0.868497888605356482827346553676761686801910400390625;0.58538485022635367016619056812487542629241943359375;0.1846656623063089586178620038481312803924083709716796875;-0.174582270011368889672809245894313789904117584228515625;-0.282588982003712685386886960259289480745792388916015625;0.89575950816956340094776578553137369453907012939453125;0.86405861882764878334484137667459435760974884033203125;0.017029546543922469137299913199967704713344573974609375;0.25296881217061983893046317461994476616382598876953125]
      mask Display: e = 0.06;c1 = [120 150 230]/255;c2 = ([120 150 230]+0)/383;c3 = ([120 150 230]+128)/383;patch([0 1 1 0],[0 0 1 1],c1);patch([0 1 1 1-e 1-e 0+e],[0 0 1 1-e 0+e 0+e],c2);patch([0 0 1 1-e 0+e 0+e],[0 1 1 1-e 1-e 0+e],c3);plot([0 1 1 0 0],[0 0 1 1 0]);disp('Weights');
  "IW{1,1}(47,:)'" : Constant  Value=[1.2929116250348295924510466647916473448276519775390625;0.58477014730587317803411906425026245415210723876953125;-0.0456022473496724700670057472962071187794208526611328125;-0.673895652110614751251205234439112246036529541015625;-0.4759887958912194516614135864074341952800750732421875;0.0270687792447638249371255625419507850892841815948486328125;-0.729454793070132279098061189870350062847137451171875;-0.72752681867528157244606745734927244484424591064453125;0.69137772322951873693597235615015961229801177978515625;1.1765984631733197307568161704693920910358428955078125]
      mask Display: e = 0.06;c1 = [120 150 230]/255;c2 = ([120 150 230]+0)/383;c3 = ([120 150 230]+128)/383;patch([0 1 1 0],[0 0 1 1],c1);patch([0 1 1 1-e 1-e 0+e],[0 0 1 1-e 0+e 0+e],c2);patch([0 0 1 1-e 0+e 0+e],[0 1 1 1-e 1-e 0+e],c3);plot([0 1 1 0 0],[0 0 1 1 0]);disp('Weights');
  "IW{1,1}(48,:)'" : Constant  Value=[0.1866041448656747814283107800292782485485076904296875;-0.6637375811264847325077198547660373151302337646484375;-0.376853697134713894190127803085488267242908477783203125;-0.2142085553795058938675310855614952743053436279296875;0.5642490714998513734457219470641575753688812255859375;0.53840978627730706751464140324969775974750518798828125;-0.0838722116200072143055166407066280953586101531982421875;-0.2346311651696332545302681182874948717653751373291015625;-1.11938770355998684635778772644698619842529296875;-0.221101591652355822237296933963079936802387237548828125]
      mask Display: e = 0.06;c1 = [120 150 230]/255;c2 = ([120 150 230]+0)/383;c3 = ([120 150 230]+128)/383;patch([0 1 1 0],[0 0 1 1],c1);patch([0 1 1 1-e 1-e 0+e],[0 0 1 1-e 0+e 0+e],c2);patch([0 0 1 1-e 0+e 0+e],[0 1 1 1-e 1-e 0+e],c3);plot([0 1 1 0 0],[0 0 1 1 0]);disp('Weights');
  "IW{1,1}(49,:)'" : Constant  Value=[0.69083203153578109922960948097170330584049224853515625;0.5097001043066342607090746241738088428974151611328125;-0.99973074720492949296613005571998655796051025390625;0.8732003616760557473952530926908366382122039794921875;0.043381490927760966991311164520084275864064693450927734375;0.504865936027117268025676821707747876644134521484375;0.030371661887866586992945627798690111376345157623291015625;-0.7373376959694664112276996092987246811389923095703125;-0.53608714377858890376415956779965199530124664306640625;-0.46273920351172825871088889471138827502727508544921875]
      mask Display: e = 0.06;c1 = [120 150 230]/255;c2 = ([120 150 230]+0)/383;c3 = ([120 150 230]+128)/383;patch([0 1 1 0],[0 0 1 1],c1);patch([0 1 1 1-e 1-e 0+e],[0 0 1 1-e 0+e 0+e],c2);patch([0 0 1 1-e 0+e 0+e],[0 1 1 1-e 1-e 0+e],c3);plot([0 1 1 0 0],[0 0 1 1 0]);disp('Weights');
  "IW{1,1}(5,:)'" : Constant  Value=[1.23833657921459217021720178308896720409393310546875;-0.6804740059077023506262094088015146553516387939453125;0.348275208676442626920533029988291673362255096435546875;-0.2038260437657128110178206270575174130499362945556640625;0.868138682045128007302992045879364013671875;0.416976148530420032134458097061724402010440826416015625;1.034357969161415535808146159979514777660369873046875;-0.5911673179391361276913130495813675224781036376953125;0.004400558649420328871659791047932230867445468902587890625;-0.330994048991054834463199085803353227674961090087890625]
      mask Display: e = 0.06;c1 = [120 150 230]/255;c2 = ([120 150 230]+0)/383;c3 = ([120 150 230]+128)/383;patch([0 1 1 0],[0 0 1 1],c1);patch([0 1 1 1-e 1-e 0+e],[0 0 1 1-e 0+e 0+e],c2);patch([0 0 1 1-e 0+e 0+e],[0 1 1 1-e 1-e 0+e],c3);plot([0 1 1 0 0],[0 0 1 1 0]);disp('Weights');
  "IW{1,1}(50,:)'" : Constant  Value=[0.56338707535445287089004295921768061816692352294921875;0.306014780762460747443043374005355872213840484619140625;1.0126509598365165398803355856216512620449066162109375;0.269959643686441819188104318527621217072010040283203125;-0.933114655235259160548366708098910748958587646484375;0.281996367950434201343767881553503684699535369873046875;0.356821884158129265518510919719119556248188018798828125;-0.32935116811230902289509003821876831352710723876953125;0.52467821714996232262961939341039396822452545166015625;1.03103578563925868394335338962264358997344970703125]
      mask Display: e = 0.06;c1 = [120 150 230]/255;c2 = ([120 150 230]+0)/383;c3 = ([120 150 230]+128)/383;patch([0 1 1 0],[0 0 1 1],c1);patch([0 1 1 1-e 1-e 0+e],[0 0 1 1-e 0+e 0+e],c2);patch([0 0 1 1-e 0+e 0+e],[0 1 1 1-e 1-e 0+e],c3);plot([0 1 1 0 0],[0 0 1 1 0]);disp('Weights');
  "IW{1,1}(6,:)'" : Constant  Value=[-0.66488904352448374712736267611035145819187164306640625;-0.715195894839907975182313748518936336040496826171875;0.1889900203042807202979957992283743806183338165283203125;-0.89996202970237904050776478470652364194393157958984375;0.841521303483980798176844473346136510372161865234375;-0.9794122971865910631805718367104418575763702392578125;-0.266873950080782018634550922797643579542636871337890625;-0.87329180815248264035943748240242712199687957763671875;0.39737648923651669452539181293104775249958038330078125;-1.15312173817929863872677742619998753070831298828125]
      mask Display: e = 0.06;c1 = [120 150 230]/255;c2 = ([120 150 230]+0)/383;c3 = ([120 150 230]+128)/383;patch([0 1 1 0],[0 0 1 1],c1);patch([0 1 1 1-e 1-e 0+e],[0 0 1 1-e 0+e 0+e],c2);patch([0 0 1 1-e 0+e 0+e],[0 1 1 1-e 1-e 0+e],c3);plot([0 1 1 0 0],[0 0 1 1 0]);disp('Weights');
  "IW{1,1}(7,:)'" : Constant  Value=[-0.7680361484884563605390894736046902835369110107421875;-1.101657102547032085482214824878610670566558837890625;-1.2973469958107097799171469887369312345981597900390625;-0.164363754453885679840396960571524687111377716064453125;0.428580095901827273774387094817939214408397674560546875;0.625419008191822722864117167773656547069549560546875;1.1884506064361379795712991835898719727993011474609375;-0.718003398872283593590282180230133235454559326171875;0.132525228666937999744135368018760345876216888427734375;-0.05786126405522180882190497186456923373043537139892578125]
      mask Display: e = 0.06;c1 = [120 150 230]/255;c2 = ([120 150 230]+0)/383;c3 = ([120 150 230]+128)/383;patch([0 1 1 0],[0 0 1 1],c1);patch([0 1 1 1-e 1-e 0+e],[0 0 1 1-e 0+e 0+e],c2);patch([0 0 1 1-e 0+e 0+e],[0 1 1 1-e 1-e 0+e],c3);plot([0 1 1 0 0],[0 0 1 1 0]);disp('Weights');
  "IW{1,1}(8,:)'" : Constant  Value=[0.3938375111045642196216931552044115960597991943359375;1.449581428143809080921755594317801296710968017578125;1.3049824409334267460991441112128086388111114501953125;0.56135899636125052847290817226166836917400360107421875;0.74516884563171803534942227997817099094390869140625;0.92272461333024946572578528503072448074817657470703125;-0.880395327718470621647384177776984870433807373046875;0.75718609781109524892173112675664015114307403564453125;-0.0819571268991821921812146456431946717202663421630859375;1.130688134597971128414428676478564739227294921875]
      mask Display: e = 0.06;c1 = [120 150 230]/255;c2 = ([120 150 230]+0)/383;c3 = ([120 150 230]+128)/383;patch([0 1 1 0],[0 0 1 1],c1);patch([0 1 1 1-e 1-e 0+e],[0 0 1 1-e 0+e 0+e],c2);patch([0 0 1 1-e 0+e 0+e],[0 1 1 1-e 1-e 0+e],c3);plot([0 1 1 0 0],[0 0 1 1 0]);disp('Weights');
  "IW{1,1}(9,:)'" : Constant  Value=[0.434844088844839105068018625388504005968570709228515625;-0.037919442056675932428699837828389718197286128997802734375;-0.042526799505366315312659963865371537394821643829345703125;0.76652211966888039729184356474434025585651397705078125;-0.60657017131881152405270540839410386979579925537109375;-0.63849617420858362226709914466482587158679962158203125;-0.6126194108765272705596771629643626511096954345703125;0.4547044441193179853399897183408029377460479736328125;-1.529203934171339707148717934614978730678558349609375;-0.52550878398265832291968990830355323851108551025390625]
      mask Display: e = 0.06;c1 = [120 150 230]/255;c2 = ([120 150 230]+0)/383;c3 = ([120 150 230]+128)/383;patch([0 1 1 0],[0 0 1 1],c1);patch([0 1 1 1-e 1-e 0+e],[0 0 1 1-e 0+e 0+e],c2);patch([0 0 1 1-e 0+e 0+e],[0 1 1 1-e 1-e 0+e],c3);plot([0 1 1 0 0],[0 0 1 1 0]);disp('Weights');
  Mux : Mux  Inputs=50
      mask Display: e = 0.06;c1 = [120 150 230]/255;c2 = ([120 150 230]+0)/383;c3 = ([120 150 230]+128)/383;patch([0 1 1 0],[0 0 1 1],c1);patch([0 1 1 1-e 1-e 0+e],[0 0 1 1-e 0+e 0+e],c2);patch([0 0 1 1-e 0+e 0+e],[0 1 1 1-e 1-e 0+e],c3);plot([0 1 1 0 0],[0 0 1 1 0]);disp('Mux');
  dotprod{1..50} (50 alike) : neural/Weight Functions/dotprod
  "iz{1,1}" : Outport
      mask Display: e = 0.06;c1 = [120 230 180]/255;c2 = ([120 230 180]+0)/(256+128);c3 = ([120 230 180]+128)/(256+128);patch([0 1 1 0],[0 0 1 1],c1);patch([0 1 1 1-e 1-e 0+e],[0 0 1 1-e 0+e 0+e],c2);patch([0 0 1 1-e 0+e 0+e],[0 1 1 1-e 1-e 0+e],c3);plot([0 1 1 0 0],[0 0 1 1 0]);
  wires:
  "IW{1,1}(1,:)'"/1 -> dotprod1/1
  "pd{1,1}"/1 -> dotprod1/2, dotprod2/2, dotprod3/2, dotprod4/2, dotprod5/2, dotprod6/2, dotprod7/2, dotprod8/2, dotprod9/2, dotprod10/2, dotprod11/2, dotprod12/2, dotprod13/2, dotprod14/2, dotprod15/2, dotprod16/2, dotprod17/2, dotprod18/2, dotprod19/2, dotprod20/2, dotprod21/2, dotprod22/2, dotprod23/2, dotprod24/2, dotprod25/2, dotprod26/2, dotprod27/2, dotprod28/2, dotprod29/2, dotprod30/2, dotprod31/2, dotprod32/2, dotprod33/2, dotprod34/2, dotprod35/2, dotprod36/2, dotprod37/2, dotprod38/2, dotprod39/2, dotprod40/2, dotprod41/2, dotprod42/2, dotprod43/2, dotprod44/2, dotprod45/2, dotprod46/2, dotprod47/2, dotprod48/2, dotprod49/2, dotprod50/2
  dotprod1/1 -> Mux/1
  "IW{1,1}(2,:)'"/1 -> dotprod2/1
  dotprod2/1 -> Mux/2
  "IW{1,1}(3,:)'"/1 -> dotprod3/1
  dotprod3/1 -> Mux/3
  "IW{1,1}(4,:)'"/1 -> dotprod4/1
  dotprod4/1 -> Mux/4
  "IW{1,1}(5,:)'"/1 -> dotprod5/1
  dotprod5/1 -> Mux/5
  "IW{1,1}(6,:)'"/1 -> dotprod6/1
  dotprod6/1 -> Mux/6
  "IW{1,1}(7,:)'"/1 -> dotprod7/1
  dotprod7/1 -> Mux/7
  "IW{1,1}(8,:)'"/1 -> dotprod8/1
  dotprod8/1 -> Mux/8
  "IW{1,1}(9,:)'"/1 -> dotprod9/1
  dotprod9/1 -> Mux/9
  "IW{1,1}(10,:)'"/1 -> dotprod10/1
  dotprod10/1 -> Mux/10
  "IW{1,1}(11,:)'"/1 -> dotprod11/1
  dotprod11/1 -> Mux/11
  "IW{1,1}(12,:)'"/1 -> dotprod12/1
  dotprod12/1 -> Mux/12
  "IW{1,1}(13,:)'"/1 -> dotprod13/1
  dotprod13/1 -> Mux/13
  "IW{1,1}(14,:)'"/1 -> dotprod14/1
  dotprod14/1 -> Mux/14
  "IW{1,1}(15,:)'"/1 -> dotprod15/1
  dotprod15/1 -> Mux/15
  "IW{1,1}(16,:)'"/1 -> dotprod16/1
  dotprod16/1 -> Mux/16
  "IW{1,1}(17,:)'"/1 -> dotprod17/1
  dotprod17/1 -> Mux/17
  "IW{1,1}(18,:)'"/1 -> dotprod18/1
  dotprod18/1 -> Mux/18
  "IW{1,1}(19,:)'"/1 -> dotprod19/1
  dotprod19/1 -> Mux/19
  "IW{1,1}(20,:)'"/1 -> dotprod20/1
  dotprod20/1 -> Mux/20
  "IW{1,1}(21,:)'"/1 -> dotprod21/1
  dotprod21/1 -> Mux/21
  "IW{1,1}(22,:)'"/1 -> dotprod22/1
  dotprod22/1 -> Mux/22
  "IW{1,1}(23,:)'"/1 -> dotprod23/1
  dotprod23/1 -> Mux/23
  "IW{1,1}(24,:)'"/1 -> dotprod24/1
  dotprod24/1 -> Mux/24
  "IW{1,1}(25,:)'"/1 -> dotprod25/1
  dotprod25/1 -> Mux/25
  "IW{1,1}(26,:)'"/1 -> dotprod26/1
  dotprod26/1 -> Mux/26
  "IW{1,1}(27,:)'"/1 -> dotprod27/1
  dotprod27/1 -> Mux/27
  "IW{1,1}(28,:)'"/1 -> dotprod28/1
  dotprod28/1 -> Mux/28
  "IW{1,1}(29,:)'"/1 -> dotprod29/1
  dotprod29/1 -> Mux/29
  "IW{1,1}(30,:)'"/1 -> dotprod30/1
  dotprod30/1 -> Mux/30
  "IW{1,1}(31,:)'"/1 -> dotprod31/1
  dotprod31/1 -> Mux/31
  "IW{1,1}(32,:)'"/1 -> dotprod32/1
  dotprod32/1 -> Mux/32
  "IW{1,1}(33,:)'"/1 -> dotprod33/1
  dotprod33/1 -> Mux/33
  "IW{1,1}(34,:)'"/1 -> dotprod34/1
  dotprod34/1 -> Mux/34
  "IW{1,1}(35,:)'"/1 -> dotprod35/1
  dotprod35/1 -> Mux/35
  "IW{1,1}(36,:)'"/1 -> dotprod36/1
  dotprod36/1 -> Mux/36
  "IW{1,1}(37,:)'"/1 -> dotprod37/1
  dotprod37/1 -> Mux/37
  "IW{1,1}(38,:)'"/1 -> dotprod38/1
  dotprod38/1 -> Mux/38
  "IW{1,1}(39,:)'"/1 -> dotprod39/1
  dotprod39/1 -> Mux/39
  "IW{1,1}(40,:)'"/1 -> dotprod40/1
  dotprod40/1 -> Mux/40
  "IW{1,1}(41,:)'"/1 -> dotprod41/1
  dotprod41/1 -> Mux/41
  "IW{1,1}(42,:)'"/1 -> dotprod42/1
  dotprod42/1 -> Mux/42
  "IW{1,1}(43,:)'"/1 -> dotprod43/1
  dotprod43/1 -> Mux/43
  "IW{1,1}(44,:)'"/1 -> dotprod44/1
  dotprod44/1 -> Mux/44
  "IW{1,1}(45,:)'"/1 -> dotprod45/1
  dotprod45/1 -> Mux/45
  "IW{1,1}(46,:)'"/1 -> dotprod46/1
  dotprod46/1 -> Mux/46
  "IW{1,1}(47,:)'"/1 -> dotprod47/1
  dotprod47/1 -> Mux/47
  "IW{1,1}(48,:)'"/1 -> dotprod48/1
  dotprod48/1 -> Mux/48
  "IW{1,1}(49,:)'"/1 -> dotprod49/1
  dotprod49/1 -> Mux/49
  "IW{1,1}(50,:)'"/1 -> dotprod50/1
  dotprod50/1 -> Mux/50
  Mux/1 -> "iz{1,1}"/1
